simulink model "sampleModel153_pp_1136_1"  (R2021a)
settings: Solver=VariableStepAuto  StartTime=0.0  StopTime=10.0  RelTol=1e-3
undefined symbols (not defined in the file or in its folder): DiscIntNeverNeededParam, magnitude, Newton, Raphson
libraries: simulink x48, pid_lib x19
(part 3 of 3)

== system sampleModel153_pp_1136_1/cfblk65/cfblk5 ==
  cfblk1 : Inport
  cfblk9 : Inport  Port=2
  cfblk10 : Inport  Port=3
  cfblk11 : Inport  Port=4
  cfblk3 : DiscreteTransferFcn  SampleTime=1
  cfblk4 : DiscreteStateSpace
  cfblk5 : Sum  Inputs=|++
  cfblk6 : simulink/Math Operations/Slider Gain  gain=1  low=0  high=2
  cfblk7 : Constant  Value=[-650905295.845550]  SampleTime=1
  cfblk8 : Constant  Value=[-876645874.250106]  SampleTime=1
  cfblk2 : Outport
  cfblk12 : Outport  Port=2
  cfblk13 : Outport  Port=3
  wires:
  cfblk9/1 -> cfblk6/1
  cfblk5/1 -> cfblk12/1
  cfblk7/1 -> cfblk4/1
  cfblk3/1 -> cfblk5/1
  cfblk10/1 -> cfblk3/1
  cfblk8/1 -> cfblk2/1
  cfblk6/1 -> cfblk5/2
  cfblk11/1 -> cfblk13/1

== system sampleModel153_pp_1136_1/cfblk66/cfblk10 ==
  cfblk1 : Inport
  cfblk10 : Inport  Port=2
  cfblk11 : Inport  Port=3
  cfblk12 : Delay  SampleTime=1
  cfblk3 : Trigonometry
  cfblk4 : Sum  Inputs=+
  cfblk5 : Sin  TimeSource=Use external signal  SampleTime=0
  cfblk6 : simulink/Math Operations/MinMax Running Resettable  Function=min  vinit=0.0
  cfblk7 : Product  Inputs=**
  cfblk8 : simulink/Math Operations/MinMax Running Resettable  Function=min  vinit=0.0
  cfblk9 : Constant  Value=[628804985.554097]  SampleTime=1
  cfblk2 : Outport
  wires:
  cfblk6/1 -> cfblk8/1
  cfblk10/1 -> cfblk2/1
  cfblk9/1 -> cfblk3/1
  cfblk4/1 -> cfblk5/1
  cfblk8/1 -> cfblk4/1
  cfblk11/1 -> cfblk6/1
  cfblk1/1 -> cfblk7/1
  cfblk3/1 -> cfblk7/2
  cfblk7/1 -> cfblk6/2
  cfblk5/1 -> cfblk12/1
  cfblk12/1 -> cfblk8/2

== system sampleModel153_pp_1136_1/cfblk66/cfblk11 ==
  cfblk1 : Inport
  cfblk14 : Inport  Port=2
  cfblk15 : Inport  Port=3
  cfblk10 : Constant  Value=[241437850.388805]  SampleTime=1
  cfblk11 : Constant  Value=[493359638.848883]  SampleTime=1
  cfblk12 : Constant  Value=[-115245312.659173]  SampleTime=1
  cfblk13 : Constant  Value=[44240335.987697]  SampleTime=1
  cfblk17 : Delay  SampleTime=1
  cfblk3 : DiscreteFir  SampleTime=1
  cfblk4 : pid_lib/PID Controller (2DOF)  Controller=PID  Form=Parallel  TimeDomain=Discrete-time  UseExternalTs=off  SampleTime=1  IntegratorMethod=Forward Euler  FilterMethod=Forward Euler  ControllerParametersSource=internal  P=1  I=1  D=0  UseFilter=on  N=100  b=1  c=1  TunerSelectOption=Transfer Function Based (PID Tuner App)  InitialConditionSource=internal  InitialConditionForIntegrator=0  InitialConditionForFilter=0  DifferentiatorICPrevScaledInput=0  ExternalReset=none  TrackingMode=off  Kt=1  LimitOutput=off  SatLimitsSource=internal  UpperSaturationLimit=inf  LowerSaturationLimit=-inf  LinearizeAsGain=off  AntiWindupMode=none  Kb=1  POutMin=[]  POutMax=[]  IOutMin=[]  IOutMax=[]  DOutMin=[]  DOutMax=[]  NOutMin=[]  NOutMax=[]  bOutMin=[]  bOutMax=[]  cOutMin=[]  cOutMax=[]  SumOutMin=[]  SumOutMax=[]  SaturationOutMin=[]  SaturationOutMax=[]  PParamMin=[]  PParamMax=[]  IParamMin=[]  IParamMax=[]  DParamMin=[]  DParamMax=[]  NParamMin=[]  NParamMax=[]  bParamMin=[]  bParamMax=[]  cParamMin=[]  cParamMax=[]  KbParamMin=[]  KbParamMax=[]  KtParamMin=[]  KtParamMax=[]  KbOutMin=[]  KbOutMax=[]  KtOutMin=[]  KtOutMax=[]  IntegratorOutMin=[]  IntegratorOutMax=[]  FilterOutMin=[]  FilterOutMax=[]  SumI1OutMin=[]  SumI1OutMax=[]  SumI2OutMin=[]  SumI2OutMax=[]  SumI3OutMin=[]  SumI3OutMax=[]  SumI4OutMin=[]  SumI4OutMax=[]  SumDOutMin=[]  SumDOutMax=[]  Sum1OutMin=[]  Sum1OutMax=[]  Sum2OutMin=[]  Sum2OutMax=[]  Sum3OutMin=[]  Sum3OutMax=[]  DifferentiatorOutMin=[]  DifferentiatorOutMax=[]  FilterDiffOutCoefMin=[]  FilterDiffOutCoefMax=[]  ReciprocalOutMin=[]  ReciprocalOutMax=[]  SumDenOutMin=[]  SumDenOutMax=[]  SumNumOutMin=[]  SumNumOutMax=[]  DivideOutMin=[]  DivideOutMax=[]  UdiffTsProdOutMin=[]  UdiffTsProdOutMax=[]  NTsProdOutMin=[]  NTsProdOutMax=[]  UintegralTsProdOutMin=[]  UintegralTsProdOutMax=[]  UngainTsProdOutMin=[]  UngainTsProdOutMax=[]  IntegratorContinuousStateAttributes=''  IntegratorStateMustResolveToSignalObject=off  IntegratorRTWStateStorageClass=Auto  FilterContinuousStateAttributes=''  FilterStateMustResolveToSignalObject=off  FilterRTWStateStorageClass=Auto  ParallelPVariant=InternalParameters  IdealPVariant=Disabled  IVariant=InternalParameters  DVariant=InternalParameters  bVariant=InternalParameters  cVariant=InternalParameters  IntegratorVariant=Discrete  SatVariant=Disabled  AWVariant=Passthrough  PCopyVariant=Disabled  TRVariant=Disabled  FdbkBlocksVariant=Forward  IdealPFdbkVariant=Disabled  SatFdbkVariant=Disabled  DerivativeFilterVariant=ForwardEulerFilter  NVariant=InternalParameters  NCopyVariant=Disabled  FilterICVariant=InternalICsFilter  IntegratorICVariant=InternalICs  ExternalResetVariant=Disabled  TRSumVariant=Passthrough  SumFdbkVariant=Disabled  SumVariant=Sum_PID  TsampFilterVariant=InternalTs  TsampNgainVariant=Passthrough  TsampIntegralVariant=Passthrough  ExternalSaturationOutDataTypeStr=Inherit: Same as second input
      settings: SourceProductBaseCode=SL
  cfblk5 : Sin  TimeSource=Use external signal  SampleTime=0
  cfblk6 : Sum  Inputs=|++
  cfblk7 : Sum  Inputs=+
  cfblk8 : simulink/Math Operations/Slider Gain  gain=1  low=0  high=2
  cfblk9 : Constant  Value=[428633806.003125]  SampleTime=1
  cfblk2 : Outport
  cfblk16 : Outport  Port=2
  wires:
  cfblk14/1 -> cfblk5/1
  cfblk9/1 -> cfblk16/1
  cfblk4/1 -> cfblk6/1
  cfblk10/1 -> cfblk3/1
  cfblk13/1 -> cfblk8/1
  cfblk5/1 -> cfblk6/2
  cfblk7/1 -> cfblk2/1
  cfblk1/1 -> cfblk7/1
  cfblk15/1 -> cfblk4/1
  cfblk6/1 -> cfblk17/1
  cfblk17/1 -> cfblk4/2

== system sampleModel153_pp_1136_1/cfblk66/cfblk4 ==
  cfblk1 : Inport
  cfblk13 : Inport  Port=2
  cfblk14 : Inport  Port=3
  cfblk10 : Squeeze
  cfblk11 : Sin  TimeSource=Use external signal  SampleTime=0
  cfblk12 : Constant  Value=[-500920913.668225]  SampleTime=1
  cfblk3 : Delay  ShowEnablePort=on  SampleTime=1
      settings: InputPortMap=u0,e6
  cfblk4 : simulink/Discrete/Difference  ICPrevInput=0.0  OutMin=[]  OutMax=[]  OutDataTypeStr=Inherit: Inherit via back propagation  OutDataType=fixdt(1, 16)  OutScaling=2^-10  DoSatur=off
  cfblk5 : simulink/Discrete/Tapped Delay  vinit=0.0  samptime=-1  NumDelays=1  DelayOrder=Oldest  includeCurrent=off
  cfblk6 : pid_lib/PID Controller  Controller=PID  Form=Parallel  TimeDomain=Discrete-time  UseExternalTs=off  SampleTime=1  IntegratorMethod=Forward Euler  FilterMethod=Forward Euler  ControllerParametersSource=internal  P=1  I=1  D=0  UseFilter=on  N=100  TunerSelectOption=Transfer Function Based (PID Tuner App)  InitialConditionSource=internal  InitialConditionForIntegrator=0  InitialConditionForFilter=0  DifferentiatorICPrevScaledInput=0  ExternalReset=none  TrackingMode=off  Kt=1  LimitOutput=off  SatLimitsSource=internal  UpperSaturationLimit=inf  LowerSaturationLimit=-inf  LinearizeAsGain=off  AntiWindupMode=none  Kb=1  POutMin=[]  POutMax=[]  IOutMin=[]  IOutMax=[]  DOutMin=[]  DOutMax=[]  NOutMin=[]  NOutMax=[]  SumOutMin=[]  SumOutMax=[]  SaturationOutMin=[]  SaturationOutMax=[]  PParamMin=[]  PParamMax=[]  IParamMin=[]  IParamMax=[]  DParamMin=[]  DParamMax=[]  NParamMin=[]  NParamMax=[]  KbParamMin=[]  KbParamMax=[]  KtParamMin=[]  KtParamMax=[]  KbOutMin=[]  KbOutMax=[]  KtOutMin=[]  KtOutMax=[]  IntegratorOutMin=[]  IntegratorOutMax=[]  FilterOutMin=[]  FilterOutMax=[]  SumI1OutMin=[]  SumI1OutMax=[]  SumI2OutMin=[]  SumI2OutMax=[]  SumI3OutMin=[]  SumI3OutMax=[]  SumI4OutMin=[]  SumI4OutMax=[]  SumDOutMin=[]  SumDOutMax=[]  DifferentiatorOutMin=[]  DifferentiatorOutMax=[]  FilterDiffOutCoefMin=[]  FilterDiffOutCoefMax=[]  ReciprocalOutMin=[]  ReciprocalOutMax=[]  SumDenOutMin=[]  SumDenOutMax=[]  SumNumOutMin=[]  SumNumOutMax=[]  DivideOutMin=[]  DivideOutMax=[]  UdiffTsProdOutMin=[]  UdiffTsProdOutMax=[]  NTsProdOutMin=[]  NTsProdOutMax=[]  UintegralTsProdOutMin=[]  UintegralTsProdOutMax=[]  UngainTsProdOutMin=[]  UngainTsProdOutMax=[]  IntegratorContinuousStateAttributes=''  IntegratorStateMustResolveToSignalObject=off  IntegratorRTWStateStorageClass=Auto  FilterContinuousStateAttributes=''  FilterStateMustResolveToSignalObject=off  FilterRTWStateStorageClass=Auto  ParallelPVariant=InternalParameters  IdealPVariant=Disabled  IVariant=InternalParameters  DVariant=InternalParameters  IntegratorVariant=Discrete  SatVariant=Disabled  AWVariant=Passthrough  PCopyVariant=Disabled  TRVariant=Disabled  FdbkBlocksVariant=Forward  IdealPFdbkVariant=Disabled  SatFdbkVariant=Disabled  DerivativeFilterVariant=ForwardEulerFilter  NVariant=InternalParameters  NCopyVariant=Disabled  FilterICVariant=InternalICsFilter  IntegratorICVariant=InternalICs  ExternalResetVariant=Disabled  TRSumVariant=Passthrough  SumFdbkVariant=Disabled  SumVariant=Sum_PID  TsampFilterVariant=InternalTs  TsampNgainVariant=Passthrough  TsampIntegralVariant=Passthrough  ExternalSaturationOutDataTypeStr=Inherit: Same as second input
  cfblk7 : Product  Inputs=**
  cfblk8 : Abs
  cfblk9 : Product  Inputs=**
  cfblk2 : Outport
  cfblk15 : Outport  Port=2
  cfblk16 : Outport  Port=3
  wires:
  cfblk6/1 -> cfblk7/1, cfblk9/2
  cfblk14/1 -> cfblk7/2
  cfblk12/1 -> cfblk8/1, cfblk9/1
  cfblk10/1 -> cfblk15/1
  cfblk8/1 -> cfblk11/1
  cfblk11/1 -> cfblk5/1
  cfblk5/1 -> cfblk4/1
  cfblk9/1 -> cfblk3/1
  cfblk7/1 -> cfblk16/1
  cfblk3/1 -> cfblk10/1
  cfblk13/1 -> cfblk6/1
  cfblk1/1 -> cfblk3/2
  cfblk4/1 -> cfblk2/1

== system sampleModel153_pp_1136_1/cfblk66/cfblk5 ==
  cfblk1 : Inport
  cfblk14 : Inport  Port=2
  cfblk15 : Inport  Port=3
  cfblk10 : Sum
  cfblk11 : Math  Operator=mod  SaturateOnIntegerOverflow=on
  cfblk12 : simulink/Math Operations/MinMax Running Resettable  Function=min  vinit=0.0
  cfblk13 : Constant  Value=[132904340.070118]  SampleTime=1
  cfblk3 : simulink/Discrete/Transfer Fcn Lead or Lag  PoleZ=0.95  ZeroZ=0.75  ICPrevOutput=0.0  ICPrevInput=0.0  DoSatur=off
      settings: SourceProductBaseCode=SL
  cfblk4 : simulink/Discrete/Tapped Delay  vinit=0.0  samptime=-1  NumDelays=1  DelayOrder=Oldest  includeCurrent=off
  cfblk5 : DiscreteStateSpace
  cfblk6 : DiscreteFir  SampleTime=1
  cfblk7 : simulink/Discrete/Transfer Fcn Real Zero  ZeroZ=0.75  ICPrevInput=0.0  DoSatur=off
      settings: SourceProductBaseCode=SL
  cfblk8 : simulink/Math Operations/MinMax Running Resettable  Function=min  vinit=0.0
  cfblk9 : Gain  Gain=[881863629.132362]
  cfblk2 : Outport
  cfblk16 : Outport  Port=2
  wires:
  cfblk1/1 -> cfblk12/1
  cfblk8/1 -> cfblk12/2
  cfblk11/1 -> cfblk10/1
  cfblk10/1 -> cfblk6/1, cfblk8/2
  cfblk3/1 -> cfblk7/1
  cfblk14/1 -> cfblk16/1
  cfblk13/1 -> cfblk9/1
  cfblk15/1 -> cfblk5/1
  cfblk7/1 -> cfblk11/1
  cfblk9/1 -> cfblk4/1
  cfblk5/1 -> cfblk10/2
  cfblk12/1 -> cfblk2/1
  cfblk4/1 -> cfblk3/1, cfblk11/2
  cfblk6/1 -> cfblk8/1

== system sampleModel153_pp_1136_1/cfblk66/cfblk6 ==
  cfblk1 : Inport
  cfblk12 : Inport  Port=2
  cfblk13 : Inport  Port=3
  cfblk14 : Inport  Port=4
  cfblk15 : Inport  Port=5
  cfblk16 : Inport  Port=6
  cfblk10 : Sum  Inputs=|++
  cfblk11 : Gain  Gain=[-117552018.394374]
  cfblk3 : Assignment  DiagnosticForDimensions=Warning  IndexOptions=Index vector (dialog)  Indices=1  OutputSizes=1
  cfblk4 : Signum
  cfblk5 : Sqrt  SaturateOnIntegerOverflow=on
  cfblk6 : Sum  Inputs=+
  cfblk7 : Sum  Inputs=+-
  cfblk8 : Sqrt  SaturateOnIntegerOverflow=on
  cfblk9 : Sum  Inputs=+-
  cfblk2 : Outport
  cfblk17 : Outport  Port=2
  wires:
  cfblk5/1 -> cfblk2/1
  cfblk14/1 -> cfblk9/1
  cfblk11/1 -> cfblk17/1
  cfblk12/1 -> cfblk9/2
  cfblk6/1 -> cfblk5/1
  cfblk10/1 -> cfblk6/1
  cfblk3/1 -> cfblk8/1
  cfblk16/1 -> cfblk3/1
  cfblk15/1 -> cfblk4/1
  cfblk13/1 -> cfblk10/1
  cfblk4/1 -> cfblk3/2
  cfblk8/1 -> cfblk10/2
  cfblk7/1 -> cfblk11/1
  cfblk9/1 -> cfblk7/1
  cfblk1/1 -> cfblk7/2

== system sampleModel153_pp_1136_1/cfblk66/cfblk7 ==
  cfblk1 : Inport
  cfblk11 : Inport  Port=2
  cfblk10 : Constant  Value=[243204345.909152]  SampleTime=1
  cfblk12 : Delay  SampleTime=1
  cfblk3 : simulink/Discrete/Transfer Fcn First Order  PoleZ=0.95  ICPrevOutput=0.0  DoSatur=off
  cfblk4 : UnitDelay  HasFrameUpgradeWarning=on
  cfblk5 : DotProduct  InputSameDT=on  OutDataTypeStr=Inherit: Inherit via internal rule
  cfblk6 : simulink/Math Operations/MinMax Running Resettable  Function=min  vinit=0.0
  cfblk7 : Polyval  Coefs=[ +2.081618890e-019, -1.441693666e-014, +4.719686976e-010, -8.536869453e-006, +1.621573104e-001, -8.087801117e+001 ]
  cfblk8 : Constant  Value=[-792798481.300644]  SampleTime=1
  cfblk9 : Constant  Value=[-993572717.090175]  SampleTime=1
  cfblk2 : Outport
  wires:
  cfblk9/1 -> cfblk3/1
  cfblk5/1 -> cfblk7/1
  cfblk10/1 -> cfblk2/1
  cfblk8/1 -> cfblk6/1
  cfblk11/1 -> cfblk6/2
  cfblk1/1 -> cfblk4/1
  cfblk6/1 -> cfblk5/1
  cfblk7/1 -> cfblk12/1
  cfblk12/1 -> cfblk5/2

== system sampleModel153_pp_1136_1/cfblk66/cfblk8 ==
  cfblk1 : Inport
  cfblk12 : Inport  Port=2
  cfblk13 : Inport  Port=3
  cfblk10 : Constant  Value=[-766566152.730124]  SampleTime=1
  cfblk11 : Constant  Value=[-183317335.996785]  SampleTime=1
  cfblk3 : DiscreteStateSpace
  cfblk4 : Delay  DelayLengthSource=Input port  SampleTime=1
      settings: InputPortMap=u0,p1
  cfblk5 : DiscreteZeroPole  Poles=[0 0.5]  Gain=1
  cfblk6 : Trigonometry
  cfblk7 : Squeeze
  cfblk8 : Abs
  cfblk9 : Constant  Value=[820543727.518785]  SampleTime=1
  cfblk2 : Outport
  cfblk14 : Outport  Port=2
  cfblk15 : Outport  Port=3
  cfblk16 : Outport  Port=4
  cfblk17 : Outport  Port=5
  wires:
  cfblk11/1 -> cfblk7/1
  cfblk4/1 -> cfblk3/1
  cfblk12/1 -> cfblk16/1
  cfblk8/1 -> cfblk5/1
  cfblk1/1 -> cfblk14/1
  cfblk5/1 -> cfblk15/1
  cfblk10/1 -> cfblk6/1
  cfblk7/1 -> cfblk17/1
  cfblk6/1 -> cfblk8/1
  cfblk9/1 -> cfblk4/1
  cfblk13/1 -> cfblk4/2
  cfblk3/1 -> cfblk2/1

== system sampleModel153_pp_1136_1/cfblk66/cfblk9 ==
  cfblk1 : Inport
  cfblk11 : Inport  Port=2
  cfblk12 : Inport  Port=3
  cfblk13 : Inport  Port=4
  cfblk14 : Inport  Port=5
  cfblk15 : Inport  Port=6
  cfblk16 : Inport  Port=7
  cfblk10 : Constant  Value=[-597004541.380494]  SampleTime=1
  cfblk3 : DiscreteFir  SampleTime=1
  cfblk4 : DiscreteTransferFcn  SampleTime=1
  cfblk5 : Product
  cfblk6 : DotProduct  InputSameDT=on  OutDataTypeStr=Inherit: Inherit via internal rule
  cfblk7 : PermuteDimensions
  cfblk8 : Constant  Value=[-643096660.058099]  SampleTime=1
  cfblk9 : Constant  Value=[904919956.485073]  SampleTime=1
  cfblk2 : Outport
  cfblk17 : Outport  Port=2
  wires:
  cfblk8/1 -> cfblk3/1
  cfblk1/1 -> cfblk6/1
  cfblk11/1 -> cfblk7/1
  cfblk10/1 -> cfblk5/1
  cfblk12/1 -> cfblk2/1
  cfblk4/1 -> cfblk17/1
  cfblk13/1 -> cfblk4/1
  cfblk14/1 -> cfblk6/2
  cfblk16/1 -> cfblk5/2

== system sampleModel153_pp_1136_1/cfblk67/cfblk4 ==
  cfblk1 : Inport
  cfblk7 : Inport  Port=2
  cfblk8 : Inport  Port=3
  cfblk9 : Inport  Port=4
  cfblk10 : Inport  Port=5
  cfblk3 : DiscreteFilter  SampleTime=1
  cfblk4 : Delay  SampleTime=1
  cfblk5 : Bias  Bias=[741704835.073662]
  cfblk6 : Constant  Value=[-124343164.537120]  SampleTime=1
  cfblk2 : Outport
  cfblk11 : Outport  Port=2
  wires:
  cfblk4/1 -> cfblk5/1
  cfblk1/1 -> cfblk4/1
  cfblk9/1 -> cfblk2/1
  cfblk6/1 -> cfblk11/1
  cfblk8/1 -> cfblk3/1

== system sampleModel153_pp_1136_1/cfblk67/cfblk5 ==
  cfblk1 : Inport
  cfblk8 : Inport  Port=2
  cfblk3 : simulink/Discrete/Difference  ICPrevInput=0.0  OutMin=[]  OutMax=[]  OutDataTypeStr=Inherit: Inherit via back propagation  OutDataType=fixdt(1, 16)  OutScaling=2^-10  DoSatur=off
  cfblk4 : Squeeze
  cfblk5 : Assignment  DiagnosticForDimensions=Warning  IndexOptions=Index vector (dialog)  Indices=1  OutputSizes=1
  cfblk6 : Sum  Inputs=|++
  cfblk7 : ComplexToRealImag
  cfblk2 : Outport
  cfblk9 : Outport  Port=2
  wires:
  cfblk8/1 -> cfblk2/1
  cfblk7/1 -> cfblk4/1
  cfblk3/1 -> cfblk6/1
  cfblk1/1 -> cfblk3/1, cfblk7/1
  cfblk6/1 -> cfblk9/1
  cfblk4/1 -> cfblk5/1
  cfblk5/1 -> cfblk6/2
  cfblk7/2 -> cfblk5/2

== system sampleModel153_pp_1136_1/cfblk69/cfblk13 ==
  cfblk1 : Inport
  cfblk9 : Inport  Port=2
  cfblk10 : Inport  Port=3
  Action Port : ActionPort  ActionPortLabel=if(u1 >= 0)
  cfblk3 : Delay  ShowEnablePort=on
      settings: InputPortMap=u0,e6
  cfblk4 : DiscreteZeroPole  Poles=[0 0.5]  Gain=1  SampleTime=-1
  cfblk5 : DiscreteIntegrator  SampleTime=-1  ICPrevOutput=DiscIntNeverNeededParam  ICPrevScaledInput=DiscIntNeverNeededParam
  cfblk6 : Abs
  cfblk7 : Sum  Inputs=+-
  cfblk8 : Constant  Value=[-836885366.925876]  SampleTime=1
  cfblk2 : Outport
  wires:
  cfblk8/1 -> cfblk6/1
  cfblk7/1 -> cfblk4/1
  cfblk10/1 -> cfblk2/1
  cfblk9/1 -> cfblk5/1
  cfblk1/1 -> cfblk7/1
  cfblk4/1 -> cfblk3/1
  cfblk5/1 -> cfblk7/2
  cfblk6/1 -> cfblk3/2

== system sampleModel153_pp_1136_1/cfblk69/cfblk14 ==
  cfblk1 : Inport
  cfblk11 : Inport  Port=2
  Action Port : ActionPort  ActionPortLabel=else
  cfblk10 : Constant  Value=[-893343908.904926]  SampleTime=1
  cfblk14 : Delay
  cfblk15 : Delay
  cfblk3 : Squeeze
  cfblk4 : Sum  Inputs=+-
  cfblk5 : Sum  Inputs=+-
  cfblk6 : Gain  Gain=[38099257.245879]
  cfblk7 : Assignment  DiagnosticForDimensions=Warning  IndexOptions=Index vector (dialog)  Indices=1  OutputSizes=1
  cfblk8 : Constant  Value=[-986735929.240885]  SampleTime=1
  cfblk9 : Constant  Value=[-408781021.898472]  SampleTime=1
  cfblk2 : Outport
  cfblk12 : Outport  Port=2
  cfblk13 : Outport  Port=3
  wires:
  cfblk9/1 -> cfblk13/1
  cfblk10/1 -> cfblk4/1
  cfblk11/1 -> cfblk2/1, cfblk12/1
  cfblk5/1 -> cfblk4/2
  cfblk1/1 -> cfblk5/2
  cfblk4/1 -> cfblk7/1
  cfblk8/1 -> cfblk7/2
  cfblk3/1 -> cfblk6/1
  cfblk7/1 -> cfblk14/1
  cfblk14/1 -> cfblk5/1
  cfblk6/1 -> cfblk15/1
  cfblk15/1 -> cfblk3/1

== system sampleModel153_pp_1136_1/cfblk69/cfblk8 ==
  cfblk1 : Inport
  cfblk11 : Inport  Port=2
  cfblk10 : Constant  Value=[170417160.690933]  SampleTime=1
  cfblk3 : DiscreteStateSpace  SampleTime=-1
  cfblk4 : Delay
  cfblk5 : UnaryMinus
  cfblk6 : Signum
  cfblk7 : Product
  cfblk8 : Sqrt  Operator=rSqrt  AlgorithmType=Newton-Raphson  SaturateOnIntegerOverflow=on
  cfblk9 : Constant  Value=[-354930483.662802]  SampleTime=1
  cfblk2 : Outport
  wires:
  cfblk9/1 -> cfblk5/1
  cfblk11/1 -> cfblk6/1
  cfblk4/1 -> cfblk3/1
  cfblk6/1 -> cfblk2/1
  cfblk10/1 -> cfblk4/1
  cfblk3/1 -> cfblk7/1
  cfblk5/1 -> cfblk7/2
  cfblk1/1 -> cfblk8/1

== system sampleModel153_pp_1136_1/cfblk70/cfblk8 ==
  cfblk1 : Inport
  cfblk5 : Inport  Port=2
  cfblk6 : Inport  Port=3
  cfblk7 : Inport  Port=4
  cfblk3 : Sum  Inputs=-+
  cfblk4 : Constant  Value=[651878708.176065]  SampleTime=1
  cfblk2 : Outport
  wires:
  cfblk5/1 -> cfblk3/1
  cfblk4/1 -> cfblk3/2
  cfblk1/1 -> cfblk2/1

== system sampleModel153_pp_1136_1/cfblk58/cfblk58/cfblk7 ==
  cfblk1 : Inport
  cfblk10 : Inport  Port=2
  cfblk11 : Inport  Port=3
  cfblk12 : Inport  Port=4
  cfblk13 : Inport  Port=5
  cfblk3 : Squeeze
  cfblk4 : DotProduct  InputSameDT=on  OutDataTypeStr=Inherit: Inherit via internal rule
  cfblk5 : Sum  Inputs=+-
  cfblk6 : Sqrt  Operator=rSqrt  AlgorithmType=Newton-Raphson  SaturateOnIntegerOverflow=on
  cfblk7 : Abs
  cfblk8 : Gain  Gain=[-811579831.073638]
  cfblk9 : Constant  Value=[-423949083.993615]  SampleTime=1
  cfblk2 : Outport
  wires:
  cfblk9/1 -> cfblk4/2
  cfblk3/1 -> cfblk6/1
  cfblk7/1 -> cfblk5/2
  cfblk13/1 -> cfblk7/1
  cfblk11/1 -> cfblk2/1
  cfblk12/1 -> cfblk3/1
  cfblk6/1 -> cfblk4/1
  cfblk10/1 -> cfblk5/1
  cfblk5/1 -> cfblk8/1

== system sampleModel153_pp_1136_1/cfblk58/cfblk58/cfblk8 ==
  cfblk1 : Inport
  cfblk14 : Inport  Port=2
  cfblk15 : Inport  Port=3
  cfblk10 : Polyval  Coefs=[ +2.081618890e-019, -1.441693666e-014, +4.719686976e-010, -8.536869453e-006, +1.621573104e-001, -8.087801117e+001 ]
  cfblk11 : Signum
  cfblk12 : Constant  Value=[-112483464.536165]  SampleTime=1
  cfblk13 : Constant  Value=[-386105699.936164]  SampleTime=1
  cfblk16 : Delay  SampleTime=1
  cfblk17 : Delay  SampleTime=1
  cfblk3 : pid_lib/PID Controller (2DOF)  Controller=PID  Form=Parallel  TimeDomain=Discrete-time  UseExternalTs=off  SampleTime=1  IntegratorMethod=Forward Euler  FilterMethod=Forward Euler  ControllerParametersSource=internal  P=1  I=1  D=0  UseFilter=on  N=100  b=1  c=1  TunerSelectOption=Transfer Function Based (PID Tuner App)  InitialConditionSource=internal  InitialConditionForIntegrator=0  InitialConditionForFilter=0  DifferentiatorICPrevScaledInput=0  ExternalReset=none  TrackingMode=off  Kt=1  LimitOutput=off  SatLimitsSource=internal  UpperSaturationLimit=inf  LowerSaturationLimit=-inf  LinearizeAsGain=off  AntiWindupMode=none  Kb=1  POutMin=[]  POutMax=[]  IOutMin=[]  IOutMax=[]  DOutMin=[]  DOutMax=[]  NOutMin=[]  NOutMax=[]  bOutMin=[]  bOutMax=[]  cOutMin=[]  cOutMax=[]  SumOutMin=[]  SumOutMax=[]  SaturationOutMin=[]  SaturationOutMax=[]  PParamMin=[]  PParamMax=[]  IParamMin=[]  IParamMax=[]  DParamMin=[]  DParamMax=[]  NParamMin=[]  NParamMax=[]  bParamMin=[]  bParamMax=[]  cParamMin=[]  cParamMax=[]  KbParamMin=[]  KbParamMax=[]  KtParamMin=[]  KtParamMax=[]  KbOutMin=[]  KbOutMax=[]  KtOutMin=[]  KtOutMax=[]  IntegratorOutMin=[]  IntegratorOutMax=[]  FilterOutMin=[]  FilterOutMax=[]  SumI1OutMin=[]  SumI1OutMax=[]  SumI2OutMin=[]  SumI2OutMax=[]  SumI3OutMin=[]  SumI3OutMax=[]  SumI4OutMin=[]  SumI4OutMax=[]  SumDOutMin=[]  SumDOutMax=[]  Sum1OutMin=[]  Sum1OutMax=[]  Sum2OutMin=[]  Sum2OutMax=[]  Sum3OutMin=[]  Sum3OutMax=[]  DifferentiatorOutMin=[]  DifferentiatorOutMax=[]  FilterDiffOutCoefMin=[]  FilterDiffOutCoefMax=[]  ReciprocalOutMin=[]  ReciprocalOutMax=[]  SumDenOutMin=[]  SumDenOutMax=[]  SumNumOutMin=[]  SumNumOutMax=[]  DivideOutMin=[]  DivideOutMax=[]  UdiffTsProdOutMin=[]  UdiffTsProdOutMax=[]  NTsProdOutMin=[]  NTsProdOutMax=[]  UintegralTsProdOutMin=[]  UintegralTsProdOutMax=[]  UngainTsProdOutMin=[]  UngainTsProdOutMax=[]  IntegratorContinuousStateAttributes=''  IntegratorStateMustResolveToSignalObject=off  IntegratorRTWStateStorageClass=Auto  FilterContinuousStateAttributes=''  FilterStateMustResolveToSignalObject=off  FilterRTWStateStorageClass=Auto  ParallelPVariant=InternalParameters  IdealPVariant=Disabled  IVariant=InternalParameters  DVariant=InternalParameters  bVariant=InternalParameters  cVariant=InternalParameters  IntegratorVariant=Discrete  SatVariant=Disabled  AWVariant=Passthrough  PCopyVariant=Disabled  TRVariant=Disabled  FdbkBlocksVariant=Forward  IdealPFdbkVariant=Disabled  SatFdbkVariant=Disabled  DerivativeFilterVariant=ForwardEulerFilter  NVariant=InternalParameters  NCopyVariant=Disabled  FilterICVariant=InternalICsFilter  IntegratorICVariant=InternalICs  ExternalResetVariant=Disabled  TRSumVariant=Passthrough  SumFdbkVariant=Disabled  SumVariant=Sum_PID  TsampFilterVariant=InternalTs  TsampNgainVariant=Passthrough  TsampIntegralVariant=Passthrough  ExternalSaturationOutDataTypeStr=Inherit: Same as second input
      settings: SourceProductBaseCode=SL
  cfblk4 : pid_lib/PID Controller (2DOF)  Controller=PID  Form=Parallel  TimeDomain=Discrete-time  UseExternalTs=off  SampleTime=1  IntegratorMethod=Forward Euler  FilterMethod=Forward Euler  ControllerParametersSource=internal  P=1  I=1  D=0  UseFilter=on  N=100  b=1  c=1  TunerSelectOption=Transfer Function Based (PID Tuner App)  InitialConditionSource=internal  InitialConditionForIntegrator=0  InitialConditionForFilter=0  DifferentiatorICPrevScaledInput=0  ExternalReset=none  TrackingMode=off  Kt=1  LimitOutput=off  SatLimitsSource=internal  UpperSaturationLimit=inf  LowerSaturationLimit=-inf  LinearizeAsGain=off  AntiWindupMode=none  Kb=1  POutMin=[]  POutMax=[]  IOutMin=[]  IOutMax=[]  DOutMin=[]  DOutMax=[]  NOutMin=[]  NOutMax=[]  bOutMin=[]  bOutMax=[]  cOutMin=[]  cOutMax=[]  SumOutMin=[]  SumOutMax=[]  SaturationOutMin=[]  SaturationOutMax=[]  PParamMin=[]  PParamMax=[]  IParamMin=[]  IParamMax=[]  DParamMin=[]  DParamMax=[]  NParamMin=[]  NParamMax=[]  bParamMin=[]  bParamMax=[]  cParamMin=[]  cParamMax=[]  KbParamMin=[]  KbParamMax=[]  KtParamMin=[]  KtParamMax=[]  KbOutMin=[]  KbOutMax=[]  KtOutMin=[]  KtOutMax=[]  IntegratorOutMin=[]  IntegratorOutMax=[]  FilterOutMin=[]  FilterOutMax=[]  SumI1OutMin=[]  SumI1OutMax=[]  SumI2OutMin=[]  SumI2OutMax=[]  SumI3OutMin=[]  SumI3OutMax=[]  SumI4OutMin=[]  SumI4OutMax=[]  SumDOutMin=[]  SumDOutMax=[]  Sum1OutMin=[]  Sum1OutMax=[]  Sum2OutMin=[]  Sum2OutMax=[]  Sum3OutMin=[]  Sum3OutMax=[]  DifferentiatorOutMin=[]  DifferentiatorOutMax=[]  FilterDiffOutCoefMin=[]  FilterDiffOutCoefMax=[]  ReciprocalOutMin=[]  ReciprocalOutMax=[]  SumDenOutMin=[]  SumDenOutMax=[]  SumNumOutMin=[]  SumNumOutMax=[]  DivideOutMin=[]  DivideOutMax=[]  UdiffTsProdOutMin=[]  UdiffTsProdOutMax=[]  NTsProdOutMin=[]  NTsProdOutMax=[]  UintegralTsProdOutMin=[]  UintegralTsProdOutMax=[]  UngainTsProdOutMin=[]  UngainTsProdOutMax=[]  IntegratorContinuousStateAttributes=''  IntegratorStateMustResolveToSignalObject=off  IntegratorRTWStateStorageClass=Auto  FilterContinuousStateAttributes=''  FilterStateMustResolveToSignalObject=off  FilterRTWStateStorageClass=Auto  ParallelPVariant=InternalParameters  IdealPVariant=Disabled  IVariant=InternalParameters  DVariant=InternalParameters  bVariant=InternalParameters  cVariant=InternalParameters  IntegratorVariant=Discrete  SatVariant=Disabled  AWVariant=Passthrough  PCopyVariant=Disabled  TRVariant=Disabled  FdbkBlocksVariant=Forward  IdealPFdbkVariant=Disabled  SatFdbkVariant=Disabled  DerivativeFilterVariant=ForwardEulerFilter  NVariant=InternalParameters  NCopyVariant=Disabled  FilterICVariant=InternalICsFilter  IntegratorICVariant=InternalICs  ExternalResetVariant=Disabled  TRSumVariant=Passthrough  SumFdbkVariant=Disabled  SumVariant=Sum_PID  TsampFilterVariant=InternalTs  TsampNgainVariant=Passthrough  TsampIntegralVariant=Passthrough  ExternalSaturationOutDataTypeStr=Inherit: Same as second input
      settings: SourceProductBaseCode=SL
  cfblk5 : Delay  ShowEnablePort=on  SampleTime=1
      settings: InputPortMap=u0,e6
  cfblk6 : simulink/Discrete/Transfer Fcn Lead or Lag  PoleZ=0.95  ZeroZ=0.75  ICPrevOutput=0.0  ICPrevInput=0.0  DoSatur=off
      settings: SourceProductBaseCode=SL
  cfblk7 : DiscreteFilter  SampleTime=1
  cfblk8 : DiscreteFir  SampleTime=1
  cfblk9 : Delay  ShowEnablePort=on  SampleTime=1
      settings: InputPortMap=u0,e6
  cfblk2 : Outport
  wires:
  cfblk17/1 -> cfblk4/2
  cfblk5/1 -> cfblk17/1
  cfblk16/1 -> cfblk3/2
  cfblk9/1 -> cfblk16/1
  cfblk4/1 -> cfblk11/1
  cfblk7/1 -> cfblk8/1
  cfblk6/1 -> cfblk9/2
  cfblk10/1 -> cfblk9/1
  cfblk14/1 -> cfblk6/1
  cfblk8/1 -> cfblk10/1
  cfblk12/1 -> cfblk4/1
  cfblk1/1 -> cfblk2/1
  cfblk3/1 -> cfblk7/1
  cfblk13/1 -> cfblk5/2
  cfblk11/1 -> cfblk5/1
  cfblk15/1 -> cfblk3/1

== system sampleModel153_pp_1136_1/cfblk58/cfblk58/cfblk9 ==
  cfblk1 : Inport
  cfblk8 : Inport  Port=2
  cfblk9 : Inport  Port=3
  cfblk10 : Inport  Port=4
  cfblk3 : Assignment  DiagnosticForDimensions=Warning  IndexOptions=Index vector (dialog)  Indices=1  OutputSizes=1
  cfblk4 : Assignment  DiagnosticForDimensions=Warning  IndexOptions=Index vector (dialog)  Indices=1  OutputSizes=1
  cfblk5 : Bias  Bias=[917769055.319509]
  cfblk6 : Rounding
  cfblk7 : Constant  Value=[-150653421.188522]  SampleTime=1
  cfblk2 : Outport
  cfblk11 : Outport  Port=2
  wires:
  cfblk6/1 -> cfblk3/2
  cfblk1/1 -> cfblk3/1
  cfblk9/1 -> cfblk6/1
  cfblk10/1 -> cfblk11/1
  cfblk8/1 -> cfblk4/2
  cfblk4/1 -> cfblk5/1
  cfblk3/1 -> cfblk2/1
  cfblk7/1 -> cfblk4/1
